simulink model "open_model"  (R2021b)
settings: Solver=ode45  StartTime=0.0  StopTime=3600*60*24  RelTol=1e-6
values from neighbouring files (symbols this model uses):
  alpha = 3.7541    [Parameters.m]
  beta = beta/(24*60*60)    (= 1.57476851852e-05)    [Parameters.m]
  dI = dI/(24*60*60)    (= 1.15740740741e-06)    [Parameters.m]
  dV = dV/(24*60*60)    (= 2.13148148148e-05)    [Parameters.m]
  I0 = 0    [Parameters.m]
  L = 936.4293    [Parameters.m]
  r = r/(24*60*60)    (= 6.97916666667e-07)    [Parameters.m]
  S0 = 128.1481    [Parameters.m]
  V0 = 0    [Parameters.m]
undefined symbols (not defined in the file or in its folder): sigbuilder_block
settings Model: Creator=zceexc1  LastModifiedBy=chenx
settings DebuggingCC: UnconnectedInputMsg=none  UnconnectedOutputMsg=none  UnconnectedLineMsg=none
settings RTWCC: DLArmComputeVersion=20.02.1

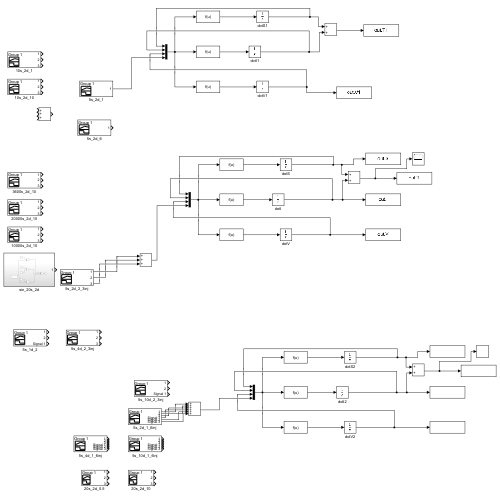
[thumbnail: Simulink's stored preview of the top-level diagram]
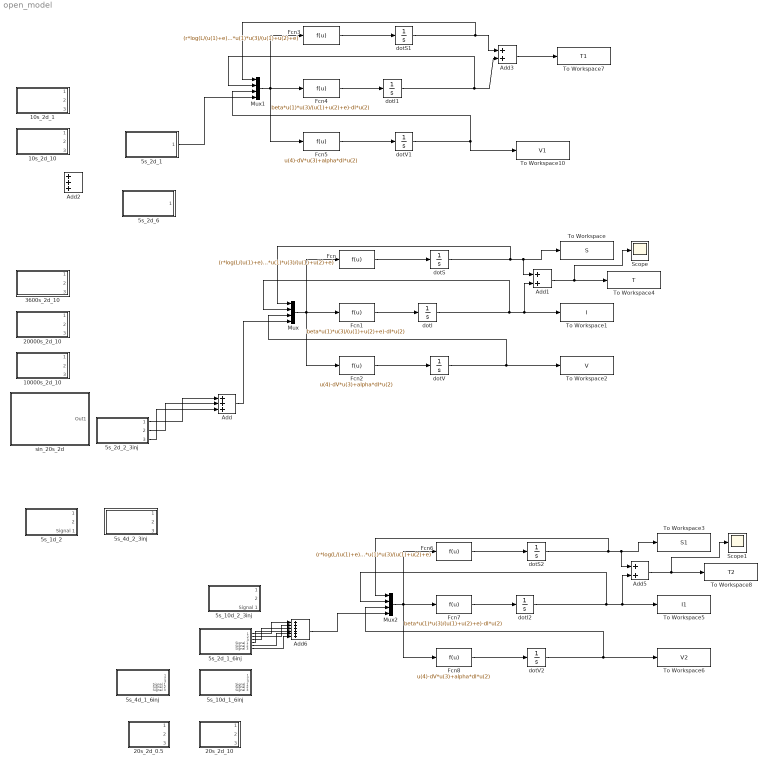
== system open_model ==
  10000s_2d_10 : Subsystem  Tag=STV Subsys  LoadFcn=sigbuilder_block('load');  StartFcn=sigbuilder_block('start');  StopFcn=sigbuilder_block('stop');  ClipboardFcn=sigbuilder_block('clipboard');  mask(Sigbuilder block){tuvar=[0:10]}
      mask help: Simulink:masks:SigbuilderBlock_MD
      mask init:
      | if ~strcmp(get_param(bdroot(gcbh),'SimulationStatus'),'stopped') tuvar = sigbuilder_block('maskInit'); end
      settings: CopyFcn=sigbuilder_block('copy');  DeleteFcn=sigbuilder_block('delete');  ModelCloseFcn=sigbuilder_block('modelClose');  PreSaveFcn=sigbuilder_block('preSave');  PauseFcn=sigbuilder_block('pause');  ContinueFcn=sigbuilder_block('continue');  NameChangeFcn=sigbuilder_block('namechange');  OpenFcn=sigbuilder_block('open',[190.5 88.5 550.5 362.5 ]);  CloseFcn=sigbuilder_block('close');
      mask Display: plot(0, 0, 100, 100,[2, 2, 32, 32, 2], [68, 8, 8, 68, 68],[32, 2], [38, 38], [32, 19, 2],[53, 60, 44], [32, 17, 17, 2],[16, 16, 31, 31]);txt = getActiveGroup(gcbh);text(2, 100, txt,'verticalAlignment', 'top');
  10s_2d_1 : Subsystem  Tag=STV Subsys  LoadFcn=sigbuilder_block('load');  StartFcn=sigbuilder_block('start');  StopFcn=sigbuilder_block('stop');  ClipboardFcn=sigbuilder_block('clipboard');  mask(Sigbuilder block){tuvar=[0:10]}
      mask help: Simulink:masks:SigbuilderBlock_MD
      mask init:
      | if ~strcmp(get_param(bdroot(gcbh),'SimulationStatus'),'stopped') tuvar = sigbuilder_block('maskInit'); end
      settings: CopyFcn=sigbuilder_block('copy');  DeleteFcn=sigbuilder_block('delete');  ModelCloseFcn=sigbuilder_block('modelClose');  PreSaveFcn=sigbuilder_block('preSave');  PauseFcn=sigbuilder_block('pause');  ContinueFcn=sigbuilder_block('continue');  NameChangeFcn=sigbuilder_block('namechange');  OpenFcn=sigbuilder_block('open',[190.5 88.5 550.5 362.5 ]);  CloseFcn=sigbuilder_block('close');
      mask Display: plot(0, 0, 100, 100,[2, 2, 32, 32, 2], [68, 8, 8, 68, 68],[32, 2], [38, 38], [32, 19, 2],[53, 60, 44], [32, 17, 17, 2],[16, 16, 31, 31]);txt = getActiveGroup(gcbh);text(2, 100, txt,'verticalAlignment', 'top');
  10s_2d_10 : Subsystem  Tag=STV Subsys  LoadFcn=sigbuilder_block('load');  StartFcn=sigbuilder_block('start');  StopFcn=sigbuilder_block('stop');  ClipboardFcn=sigbuilder_block('clipboard');  mask(Sigbuilder block){tuvar=[0:10]}
      mask help: Simulink:masks:SigbuilderBlock_MD
      mask init:
      | if ~strcmp(get_param(bdroot(gcbh),'SimulationStatus'),'stopped') tuvar = sigbuilder_block('maskInit'); end
      settings: CopyFcn=sigbuilder_block('copy');  DeleteFcn=sigbuilder_block('delete');  ModelCloseFcn=sigbuilder_block('modelClose');  PreSaveFcn=sigbuilder_block('preSave');  PauseFcn=sigbuilder_block('pause');  ContinueFcn=sigbuilder_block('continue');  NameChangeFcn=sigbuilder_block('namechange');  OpenFcn=sigbuilder_block('open',[190.5 88.5 550.5 362.5 ]);  CloseFcn=sigbuilder_block('close');
      mask Display: plot(0, 0, 100, 100,[2, 2, 32, 32, 2], [68, 8, 8, 68, 68],[32, 2], [38, 38], [32, 19, 2],[53, 60, 44], [32, 17, 17, 2],[16, 16, 31, 31]);txt = getActiveGroup(gcbh);text(2, 100, txt,'verticalAlignment', 'top');
  20000s_2d_10 : Subsystem  Tag=STV Subsys  LoadFcn=sigbuilder_block('load');  StartFcn=sigbuilder_block('start');  StopFcn=sigbuilder_block('stop');  ClipboardFcn=sigbuilder_block('clipboard');  mask(Sigbuilder block){tuvar=[0:10]}
      mask help: Simulink:masks:SigbuilderBlock_MD
      mask init:
      | if ~strcmp(get_param(bdroot(gcbh),'SimulationStatus'),'stopped') tuvar = sigbuilder_block('maskInit'); end
      settings: CopyFcn=sigbuilder_block('copy');  DeleteFcn=sigbuilder_block('delete');  ModelCloseFcn=sigbuilder_block('modelClose');  PreSaveFcn=sigbuilder_block('preSave');  PauseFcn=sigbuilder_block('pause');  ContinueFcn=sigbuilder_block('continue');  NameChangeFcn=sigbuilder_block('namechange');  OpenFcn=sigbuilder_block('open',[190.5 88.5 550.5 362.5 ]);  CloseFcn=sigbuilder_block('close');
      mask Display: plot(0, 0, 100, 100,[2, 2, 32, 32, 2], [68, 8, 8, 68, 68],[32, 2], [38, 38], [32, 19, 2],[53, 60, 44], [32, 17, 17, 2],[16, 16, 31, 31]);txt = getActiveGroup(gcbh);text(2, 100, txt,'verticalAlignment', 'top');
  20s_2d_0.5 : Subsystem  Tag=STV Subsys  LoadFcn=sigbuilder_block('load');  StartFcn=sigbuilder_block('start');  StopFcn=sigbuilder_block('stop');  ClipboardFcn=sigbuilder_block('clipboard');  mask(Sigbuilder block){tuvar=[0:10]}
      mask help: Simulink:masks:SigbuilderBlock_MD
      mask init:
      | if ~strcmp(get_param(bdroot(gcbh),'SimulationStatus'),'stopped') tuvar = sigbuilder_block('maskInit'); end
      settings: CopyFcn=sigbuilder_block('copy');  DeleteFcn=sigbuilder_block('delete');  ModelCloseFcn=sigbuilder_block('modelClose');  PreSaveFcn=sigbuilder_block('preSave');  PauseFcn=sigbuilder_block('pause');  ContinueFcn=sigbuilder_block('continue');  NameChangeFcn=sigbuilder_block('namechange');  OpenFcn=sigbuilder_block('open',[190.5 88.5 550.5 362.5 ]);  CloseFcn=sigbuilder_block('close');
      mask Display: plot(0, 0, 100, 100,[2, 2, 32, 32, 2], [68, 8, 8, 68, 68],[32, 2], [38, 38], [32, 19, 2],[53, 60, 44], [32, 17, 17, 2],[16, 16, 31, 31]);txt = getActiveGroup(gcbh);text(2, 100, txt,'verticalAlignment', 'top');
  20s_2d_10 : Subsystem  Tag=STV Subsys  LoadFcn=sigbuilder_block('load');  StartFcn=sigbuilder_block('start');  StopFcn=sigbuilder_block('stop');  ClipboardFcn=sigbuilder_block('clipboard');  mask(Sigbuilder block){tuvar=[0:10]}
      mask help: Simulink:masks:SigbuilderBlock_MD
      mask init:
      | if ~strcmp(get_param(bdroot(gcbh),'SimulationStatus'),'stopped') tuvar = sigbuilder_block('maskInit'); end
      settings: CopyFcn=sigbuilder_block('copy');  DeleteFcn=sigbuilder_block('delete');  ModelCloseFcn=sigbuilder_block('modelClose');  PreSaveFcn=sigbuilder_block('preSave');  PauseFcn=sigbuilder_block('pause');  ContinueFcn=sigbuilder_block('continue');  NameChangeFcn=sigbuilder_block('namechange');  OpenFcn=sigbuilder_block('open',[190.5 88.5 550.5 362.5 ]);  CloseFcn=sigbuilder_block('close');
      mask Display: plot(0, 0, 100, 100,[2, 2, 32, 32, 2], [68, 8, 8, 68, 68],[32, 2], [38, 38], [32, 19, 2],[53, 60, 44], [32, 17, 17, 2],[16, 16, 31, 31]);txt = getActiveGroup(gcbh);text(2, 100, txt,'verticalAlignment', 'top');
  3600s_2d_10 : Subsystem  Tag=STV Subsys  LoadFcn=sigbuilder_block('load');  StartFcn=sigbuilder_block('start');  StopFcn=sigbuilder_block('stop');  ClipboardFcn=sigbuilder_block('clipboard');  mask(Sigbuilder block){tuvar=[0:10]}
      mask help: Simulink:masks:SigbuilderBlock_MD
      mask init:
      | if ~strcmp(get_param(bdroot(gcbh),'SimulationStatus'),'stopped') tuvar = sigbuilder_block('maskInit'); end
      settings: CopyFcn=sigbuilder_block('copy');  DeleteFcn=sigbuilder_block('delete');  ModelCloseFcn=sigbuilder_block('modelClose');  PreSaveFcn=sigbuilder_block('preSave');  PauseFcn=sigbuilder_block('pause');  ContinueFcn=sigbuilder_block('continue');  NameChangeFcn=sigbuilder_block('namechange');  OpenFcn=sigbuilder_block('open',[190.5 88.5 550.5 362.5 ]);  CloseFcn=sigbuilder_block('close');
      mask Display: plot(0, 0, 100, 100,[2, 2, 32, 32, 2], [68, 8, 8, 68, 68],[32, 2], [38, 38], [32, 19, 2],[53, 60, 44], [32, 17, 17, 2],[16, 16, 31, 31]);txt = getActiveGroup(gcbh);text(2, 100, txt,'verticalAlignment', 'top');
  5s_10d_1_6inj : Subsystem  Tag=STV Subsys  LoadFcn=sigbuilder_block('load');  StartFcn=sigbuilder_block('start');  StopFcn=sigbuilder_block('stop');  ClipboardFcn=sigbuilder_block('clipboard');  mask(Sigbuilder block){tuvar=[0:10]}
      mask help: Simulink:masks:SigbuilderBlock_MD
      mask init:
      | if ~strcmp(get_param(bdroot(gcbh),'SimulationStatus'),'stopped') tuvar = sigbuilder_block('maskInit'); end
      settings: CopyFcn=sigbuilder_block('copy');  DeleteFcn=sigbuilder_block('delete');  ModelCloseFcn=sigbuilder_block('modelClose');  PreSaveFcn=sigbuilder_block('preSave');  PauseFcn=sigbuilder_block('pause');  ContinueFcn=sigbuilder_block('continue');  NameChangeFcn=sigbuilder_block('namechange');  OpenFcn=sigbuilder_block('open',[190.5 88.5 550.5 362.5 ]);  CloseFcn=sigbuilder_block('close');
      mask Display: plot(0, 0, 100, 100,[2, 2, 32, 32, 2], [68, 8, 8, 68, 68],[32, 2], [38, 38], [32, 19, 2],[53, 60, 44], [32, 17, 17, 2],[16, 16, 31, 31]);txt = getActiveGroup(gcbh);text(2, 100, txt,'verticalAlignment', 'top');
  5s_10d_2_3inj : Subsystem  Tag=STV Subsys  LoadFcn=sigbuilder_block('load');  StartFcn=sigbuilder_block('start');  StopFcn=sigbuilder_block('stop');  ClipboardFcn=sigbuilder_block('clipboard');  mask(Sigbuilder block){tuvar=[0:10]}
      mask help: Simulink:masks:SigbuilderBlock_MD
      mask init:
      | if ~strcmp(get_param(bdroot(gcbh),'SimulationStatus'),'stopped') tuvar = sigbuilder_block('maskInit'); end
      settings: CopyFcn=sigbuilder_block('copy');  DeleteFcn=sigbuilder_block('delete');  ModelCloseFcn=sigbuilder_block('modelClose');  PreSaveFcn=sigbuilder_block('preSave');  PauseFcn=sigbuilder_block('pause');  ContinueFcn=sigbuilder_block('continue');  NameChangeFcn=sigbuilder_block('namechange');  OpenFcn=sigbuilder_block('open',[190.5 88.5 550.5 362.5 ]);  CloseFcn=sigbuilder_block('close');
      mask Display: plot(0, 0, 100, 100,[2, 2, 32, 32, 2], [68, 8, 8, 68, 68],[32, 2], [38, 38], [32, 19, 2],[53, 60, 44], [32, 17, 17, 2],[16, 16, 31, 31]);txt = getActiveGroup(gcbh);text(2, 100, txt,'verticalAlignment', 'top');
  5s_1d_2 : Subsystem  Tag=STV Subsys  LoadFcn=sigbuilder_block('load');  StartFcn=sigbuilder_block('start');  StopFcn=sigbuilder_block('stop');  ClipboardFcn=sigbuilder_block('clipboard');  mask(Sigbuilder block){tuvar=[0:10]}
      mask help: Simulink:masks:SigbuilderBlock_MD
      mask init:
      | if ~strcmp(get_param(bdroot(gcbh),'SimulationStatus'),'stopped') tuvar = sigbuilder_block('maskInit'); end
      settings: CopyFcn=sigbuilder_block('copy');  DeleteFcn=sigbuilder_block('delete');  ModelCloseFcn=sigbuilder_block('modelClose');  PreSaveFcn=sigbuilder_block('preSave');  PauseFcn=sigbuilder_block('pause');  ContinueFcn=sigbuilder_block('continue');  NameChangeFcn=sigbuilder_block('namechange');  OpenFcn=sigbuilder_block('open',[190.5 88.5 550.5 362.5 ]);  CloseFcn=sigbuilder_block('close');
      mask Display: plot(0, 0, 100, 100,[2, 2, 32, 32, 2], [68, 8, 8, 68, 68],[32, 2], [38, 38], [32, 19, 2],[53, 60, 44], [32, 17, 17, 2],[16, 16, 31, 31]);txt = getActiveGroup(gcbh);text(2, 100, txt,'verticalAlignment', 'top');
  5s_2d_1 : Subsystem  Tag=STV Subsys  LoadFcn=sigbuilder_block('load');  StartFcn=sigbuilder_block('start');  StopFcn=sigbuilder_block('stop');  ClipboardFcn=sigbuilder_block('clipboard');  mask(Sigbuilder block){tuvar=[0:10]}
      mask help: Simulink:masks:SigbuilderBlock_MD
      mask init:
      | if ~strcmp(get_param(bdroot(gcbh),'SimulationStatus'),'stopped') tuvar = sigbuilder_block('maskInit'); end
      settings: CopyFcn=sigbuilder_block('copy');  DeleteFcn=sigbuilder_block('delete');  ModelCloseFcn=sigbuilder_block('modelClose');  PreSaveFcn=sigbuilder_block('preSave');  PauseFcn=sigbuilder_block('pause');  ContinueFcn=sigbuilder_block('continue');  NameChangeFcn=sigbuilder_block('namechange');  OpenFcn=sigbuilder_block('open',[190.5 88.5 550.5 362.5 ]);  CloseFcn=sigbuilder_block('close');
      mask Display: plot(0, 0, 100, 100,[2, 2, 32, 32, 2], [68, 8, 8, 68, 68],[32, 2], [38, 38], [32, 19, 2],[53, 60, 44], [32, 17, 17, 2],[16, 16, 31, 31]);txt = getActiveGroup(gcbh);text(2, 100, txt,'verticalAlignment', 'top');
  5s_2d_1_6inj : Subsystem  Tag=STV Subsys  LoadFcn=sigbuilder_block('load');  StartFcn=sigbuilder_block('start');  StopFcn=sigbuilder_block('stop');  ClipboardFcn=sigbuilder_block('clipboard');  mask(Sigbuilder block){tuvar=[0:10]}
      mask help: Simulink:masks:SigbuilderBlock_MD
      mask init:
      | if ~strcmp(get_param(bdroot(gcbh),'SimulationStatus'),'stopped') tuvar = sigbuilder_block('maskInit'); end
      settings: CopyFcn=sigbuilder_block('copy');  DeleteFcn=sigbuilder_block('delete');  ModelCloseFcn=sigbuilder_block('modelClose');  PreSaveFcn=sigbuilder_block('preSave');  PauseFcn=sigbuilder_block('pause');  ContinueFcn=sigbuilder_block('continue');  NameChangeFcn=sigbuilder_block('namechange');  OpenFcn=sigbuilder_block('open',[190.5 88.5 550.5 362.5 ]);  CloseFcn=sigbuilder_block('close');
      mask Display: plot(0, 0, 100, 100,[2, 2, 32, 32, 2], [68, 8, 8, 68, 68],[32, 2], [38, 38], [32, 19, 2],[53, 60, 44], [32, 17, 17, 2],[16, 16, 31, 31]);txt = getActiveGroup(gcbh);text(2, 100, txt,'verticalAlignment', 'top');
  5s_2d_2_3inj : Subsystem  Tag=STV Subsys  LoadFcn=sigbuilder_block('load');  StartFcn=sigbuilder_block('start');  StopFcn=sigbuilder_block('stop');  ClipboardFcn=sigbuilder_block('clipboard');  mask(Sigbuilder block){tuvar=[0:10]}
      mask help: Simulink:masks:SigbuilderBlock_MD
      mask init:
      | if ~strcmp(get_param(bdroot(gcbh),'SimulationStatus'),'stopped') tuvar = sigbuilder_block('maskInit'); end
      settings: CopyFcn=sigbuilder_block('copy');  DeleteFcn=sigbuilder_block('delete');  ModelCloseFcn=sigbuilder_block('modelClose');  PreSaveFcn=sigbuilder_block('preSave');  PauseFcn=sigbuilder_block('pause');  ContinueFcn=sigbuilder_block('continue');  NameChangeFcn=sigbuilder_block('namechange');  OpenFcn=sigbuilder_block('open',[190.5 88.5 550.5 362.5 ]);  CloseFcn=sigbuilder_block('close');
      mask Display: plot(0, 0, 100, 100,[2, 2, 32, 32, 2], [68, 8, 8, 68, 68],[32, 2], [38, 38], [32, 19, 2],[53, 60, 44], [32, 17, 17, 2],[16, 16, 31, 31]);txt = getActiveGroup(gcbh);text(2, 100, txt,'verticalAlignment', 'top');
  5s_2d_6 : Subsystem  Tag=STV Subsys  LoadFcn=sigbuilder_block('load');  StartFcn=sigbuilder_block('start');  StopFcn=sigbuilder_block('stop');  ClipboardFcn=sigbuilder_block('clipboard');  mask(Sigbuilder block){tuvar=[0:10]}
      mask help: Simulink:masks:SigbuilderBlock_MD
      mask init:
      | if ~strcmp(get_param(bdroot(gcbh),'SimulationStatus'),'stopped') tuvar = sigbuilder_block('maskInit'); end
      settings: CopyFcn=sigbuilder_block('copy');  DeleteFcn=sigbuilder_block('delete');  ModelCloseFcn=sigbuilder_block('modelClose');  PreSaveFcn=sigbuilder_block('preSave');  PauseFcn=sigbuilder_block('pause');  ContinueFcn=sigbuilder_block('continue');  NameChangeFcn=sigbuilder_block('namechange');  OpenFcn=sigbuilder_block('open',[190.5 88.5 550.5 362.5 ]);  CloseFcn=sigbuilder_block('close');
      mask Display: plot(0, 0, 100, 100,[2, 2, 32, 32, 2], [68, 8, 8, 68, 68],[32, 2], [38, 38], [32, 19, 2],[53, 60, 44], [32, 17, 17, 2],[16, 16, 31, 31]);txt = getActiveGroup(gcbh);text(2, 100, txt,'verticalAlignment', 'top');
  5s_4d_1_6inj : Subsystem  Tag=STV Subsys  LoadFcn=sigbuilder_block('load');  StartFcn=sigbuilder_block('start');  StopFcn=sigbuilder_block('stop');  ClipboardFcn=sigbuilder_block('clipboard');  mask(Sigbuilder block){tuvar=[0:10]}
      mask help: Simulink:masks:SigbuilderBlock_MD
      mask init:
      | if ~strcmp(get_param(bdroot(gcbh),'SimulationStatus'),'stopped') tuvar = sigbuilder_block('maskInit'); end
      settings: CopyFcn=sigbuilder_block('copy');  DeleteFcn=sigbuilder_block('delete');  ModelCloseFcn=sigbuilder_block('modelClose');  PreSaveFcn=sigbuilder_block('preSave');  PauseFcn=sigbuilder_block('pause');  ContinueFcn=sigbuilder_block('continue');  NameChangeFcn=sigbuilder_block('namechange');  OpenFcn=sigbuilder_block('open',[190.5 88.5 550.5 362.5 ]);  CloseFcn=sigbuilder_block('close');
      mask Display: plot(0, 0, 100, 100,[2, 2, 32, 32, 2], [68, 8, 8, 68, 68],[32, 2], [38, 38], [32, 19, 2],[53, 60, 44], [32, 17, 17, 2],[16, 16, 31, 31]);txt = getActiveGroup(gcbh);text(2, 100, txt,'verticalAlignment', 'top');
  5s_4d_2_3inj : Subsystem  Tag=STV Subsys  LoadFcn=sigbuilder_block('load');  StartFcn=sigbuilder_block('start');  StopFcn=sigbuilder_block('stop');  ClipboardFcn=sigbuilder_block('clipboard');  mask(Sigbuilder block){tuvar=[0:10]}
      mask help: Simulink:masks:SigbuilderBlock_MD
      mask init:
      | if ~strcmp(get_param(bdroot(gcbh),'SimulationStatus'),'stopped') tuvar = sigbuilder_block('maskInit'); end
      settings: CopyFcn=sigbuilder_block('copy');  DeleteFcn=sigbuilder_block('delete');  ModelCloseFcn=sigbuilder_block('modelClose');  PreSaveFcn=sigbuilder_block('preSave');  PauseFcn=sigbuilder_block('pause');  ContinueFcn=sigbuilder_block('continue');  NameChangeFcn=sigbuilder_block('namechange');  OpenFcn=sigbuilder_block('open',[190.5 88.5 550.5 362.5 ]);  CloseFcn=sigbuilder_block('close');
      mask Display: plot(0, 0, 100, 100,[2, 2, 32, 32, 2], [68, 8, 8, 68, 68],[32, 2], [38, 38], [32, 19, 2],[53, 60, 44], [32, 17, 17, 2],[16, 16, 31, 31]);txt = getActiveGroup(gcbh);text(2, 100, txt,'verticalAlignment', 'top');
  Add : Sum  Inputs=+++
  Add1 : Sum
  Add2 : Sum  Inputs=+++
  Add3 : Sum
  Add5 : Sum
  Add6 : Sum  Inputs=++++++
  Fcn : Fcn  Expr=(r*log(L/(u(1)+e)))*u(1)-beta*u(1)*u(3)/(u(1)+u(2)+e)
  Fcn1 : Fcn  Expr=beta*u(1)*u(3)/(u(1)+u(2)+e)-dI*u(2)
  Fcn2 : Fcn  Expr=u(4)-dV*u(3)+alpha*dI*u(2)
  Fcn3 : Fcn  Expr=(r*log(L/(u(1)+e)))*u(1)-beta*u(1)*u(3)/(u(1)+u(2)+e)
  Fcn4 : Fcn  Expr=beta*u(1)*u(3)/(u(1)+u(2)+e)-dI*u(2)
  Fcn5 : Fcn  Expr=u(4)-dV*u(3)+alpha*dI*u(2)
  Fcn6 : Fcn  Expr=(r*log(L/(u(1)+e)))*u(1)-beta*u(1)*u(3)/(u(1)+u(2)+e)
  Fcn7 : Fcn  Expr=beta*u(1)*u(3)/(u(1)+u(2)+e)-dI*u(2)
  Fcn8 : Fcn  Expr=u(4)-dV*u(3)+alpha*dI*u(2)
  Mux : Mux
  Mux1 : Mux
  Mux2 : Mux
  Scope : Scope
  Scope1 : Scope
  To Workspace : ToWorkspace  VariableName=S  SampleTime=-1
  To Workspace1 : ToWorkspace  VariableName=I  SampleTime=-1
  To Workspace10 : ToWorkspace  VariableName=V1  SampleTime=-1
  To Workspace2 : ToWorkspace  VariableName=V  SampleTime=-1
  To Workspace3 : ToWorkspace  VariableName=S1  SampleTime=-1
  To Workspace4 : ToWorkspace  VariableName=T  SampleTime=-1
  To Workspace5 : ToWorkspace  VariableName=I1  SampleTime=-1
  To Workspace6 : ToWorkspace  VariableName=V2  SampleTime=-1
  To Workspace7 : ToWorkspace  VariableName=T1  SampleTime=-1
  To Workspace8 : ToWorkspace  VariableName=T2  SampleTime=-1
  dotI : Integrator  InitialCondition=I0
  dotI1 : Integrator  InitialCondition=I0
  dotI2 : Integrator  InitialCondition=I0
  dotS : Integrator  InitialCondition=S0
  dotS1 : Integrator  InitialCondition=S0
  dotS2 : Integrator  InitialCondition=S0
  dotV : Integrator  InitialCondition=V0
  dotV1 : Integrator  InitialCondition=V0
  dotV2 : Integrator  InitialCondition=V0
  sin_20s_2d : Subsystem
  wires:
  Fcn/1 -> dotS/1
  Fcn1/1 -> dotI/1
  Fcn2/1 -> dotV/1
  dotV/1 -> Mux/3, To Workspace2/1
  dotS/1 -> Add1/1, To Workspace/1, Mux/1
  dotI/1 -> Add1/2, To Workspace1/1, Mux/2
  Mux/1 -> Fcn1/1, Fcn/1, Fcn2/1
  Add/1 -> Mux/4
  Add1/1 -> Scope/1, To Workspace4/1
  Mux1/1 -> Fcn4/1, Fcn3/1, Fcn5/1
  dotV1/1 -> Mux1/3, To Workspace10/1
  Fcn5/1 -> dotV1/1
  Fcn4/1 -> dotI1/1
  Add3/1 -> To Workspace7/1
  dotS1/1 -> Add3/1, Mux1/1
  Fcn3/1 -> dotS1/1
  dotI1/1 -> Add3/2, Mux1/2
  Mux2/1 -> Fcn7/1, Fcn6/1, Fcn8/1
  dotV2/1 -> Mux2/3, To Workspace6/1
  Fcn8/1 -> dotV2/1
  Fcn7/1 -> dotI2/1
  Add5/1 -> Scope1/1, To Workspace8/1
  dotS2/1 -> Add5/1, To Workspace3/1, Mux2/1
  Fcn6/1 -> dotS2/1
  dotI2/1 -> Add5/2, To Workspace5/1, Mux2/2
  Add6/1 -> Mux2/4
  5s_2d_1_6inj/1(1) -> Add6/1
  5s_2d_1_6inj/2(2) -> Add6/2
  5s_2d_1_6inj/3(3) -> Add6/3
  5s_2d_1_6inj/4(Signal 1) -> Add6/4
  5s_2d_1_6inj/5(Signal 2) -> Add6/5
  5s_2d_1_6inj/6(Signal 3) -> Add6/6
  5s_2d_2_3inj/1(1) -> Add/1
  5s_2d_2_3inj/2(2) -> Add/2
  5s_2d_2_3inj/3(3) -> Add/3
  5s_2d_1/1(1) -> Mux1/4

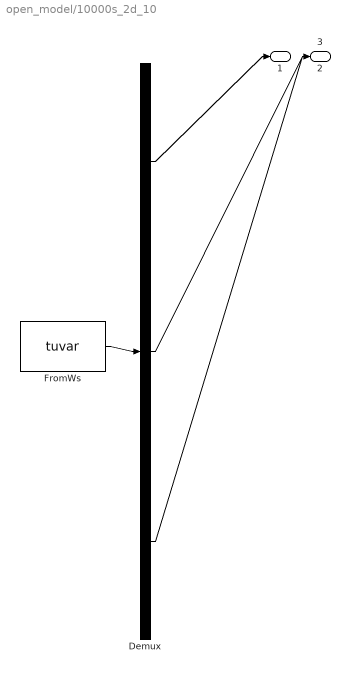
== system open_model/10000s_2d_10 ==
  Demux : Demux  Tag=STV Demux  Outputs=3
      settings: DisplayOption=none
  FromWs : FromWorkspace  Tag=STV FromWs  VariableName=tuvar
      SigBuilderData=|
      | common.afterFinalStr = 'Extrapolate'
      | common.sampleTime = 0
      | dataSet.timeRange = [0 864000]
      | dataSet.name = 'Group 1'
      | sbobj.Groups.Name = 'Group 1'
      | sbobj.Groups.Signals(1).Name = '1'
      | sbobj.Groups.Signals(1).XData = [0 10000 10000 864000]
      | sbobj.Groups.Signals(1).YData = [10 10 0 0]
      | sbobj.Groups.Signals(2).Name = '2'
      | sbobj.Groups.Signals(2).XData = [0 172800 172800 182800 182800 864000]
      | sbobj.Groups.Signals(2).YData = [0 0 10 10 0 0]
      | sbobj.Groups.Signals(3).Name = '3'
      | sbobj.Groups.Signals(3).XData = [0 345600 345600 355600 355600 864000]
      | sbobj.Groups.Signals(3).YData = [0 0 10 10 0 0]
      | sbobj.Groups.TimeRange = [0 864000]
  1 : Outport  Tag=STV Outport
  2 : Outport  Tag=STV Outport  Port=2
  3 : Outport  Tag=STV Outport  Port=3
  wires:
  Demux/1 -> 1/1
  Demux/2 -> 2/1
  Demux/3 -> 3/1
  FromWs/1 -> Demux/1

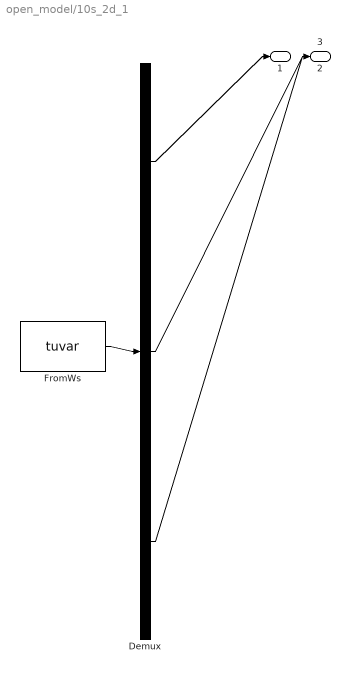
== system open_model/10s_2d_1 ==
  Demux : Demux  Tag=STV Demux  Outputs=3
      settings: DisplayOption=none
  FromWs : FromWorkspace  Tag=STV FromWs  VariableName=tuvar
      SigBuilderData=|
      | common.afterFinalStr = 'Extrapolate'
      | common.sampleTime = 0
      | dataSet.timeRange = [0 864000]
      | dataSet.name = 'Group 1'
      | sbobj.Groups.Name = 'Group 1'
      | sbobj.Groups.Signals(1).Name = '1'
      | sbobj.Groups.Signals(1).XData = [0 10 10 864000]
      | sbobj.Groups.Signals(1).YData = [1 1 0 0]
      | sbobj.Groups.Signals(2).Name = '2'
      | sbobj.Groups.Signals(2).XData = [0 172800 172800 172810 172810 864000]
      | sbobj.Groups.Signals(2).YData = [0 0 1 1 0 0]
      | sbobj.Groups.Signals(3).Name = '3'
      | sbobj.Groups.Signals(3).XData = [0 345600 345600 345610 345610 864000]
      | sbobj.Groups.Signals(3).YData = [0 0 1 1 0 0]
      | sbobj.Groups.TimeRange = [0 864000]
  1 : Outport  Tag=STV Outport
  2 : Outport  Tag=STV Outport  Port=2
  3 : Outport  Tag=STV Outport  Port=3
  wires:
  FromWs/1 -> Demux/1
  Demux/3 -> 3/1
  Demux/2 -> 2/1
  Demux/1 -> 1/1

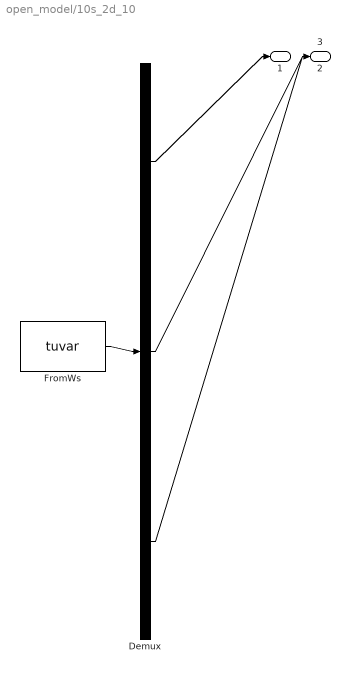
== system open_model/10s_2d_10 ==
  Demux : Demux  Tag=STV Demux  Outputs=3
      settings: DisplayOption=none
  FromWs : FromWorkspace  Tag=STV FromWs  VariableName=tuvar
      SigBuilderData=|
      | common.afterFinalStr = 'Extrapolate'
      | common.sampleTime = 0
      | dataSet.timeRange = [0 864000]
      | dataSet.name = 'Group 1'
      | sbobj.Groups.Name = 'Group 1'
      | sbobj.Groups.Signals(1).Name = '1'
      | sbobj.Groups.Signals(1).XData = [0 10 10 864000]
      | sbobj.Groups.Signals(1).YData = [10 10 0 0]
      | sbobj.Groups.Signals(2).Name = '2'
      | sbobj.Groups.Signals(2).XData = [0 172800 172800 172810 172810 864000]
      | sbobj.Groups.Signals(2).YData = [0 0 10 10 0 0]
      | sbobj.Groups.Signals(3).Name = '3'
      | sbobj.Groups.Signals(3).XData = [0 345600 345600 345610 345610 864000]
      | sbobj.Groups.Signals(3).YData = [0 0 10 10 0 0]
      | sbobj.Groups.TimeRange = [0 864000]
  1 : Outport  Tag=STV Outport
  2 : Outport  Tag=STV Outport  Port=2
  3 : Outport  Tag=STV Outport  Port=3
  wires:
  Demux/1 -> 1/1
  Demux/2 -> 2/1
  Demux/3 -> 3/1
  FromWs/1 -> Demux/1

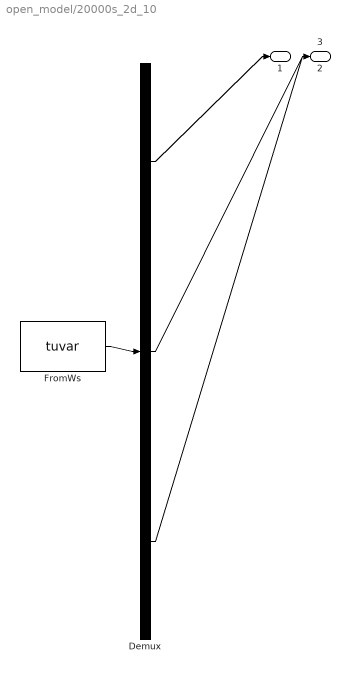
== system open_model/20000s_2d_10 ==
  Demux : Demux  Tag=STV Demux  Outputs=3
      settings: DisplayOption=none
  FromWs : FromWorkspace  Tag=STV FromWs  VariableName=tuvar
      SigBuilderData=|
      | common.afterFinalStr = 'Extrapolate'
      | common.sampleTime = 0
      | dataSet.timeRange = [0 864000]
      | dataSet.name = 'Group 1'
      | sbobj.Groups.Name = 'Group 1'
      | sbobj.Groups.Signals(1).Name = '1'
      | sbobj.Groups.Signals(1).XData = [0 20000 20000 864000]
      | sbobj.Groups.Signals(1).YData = [10 10 0 0]
      | sbobj.Groups.Signals(2).Name = '2'
      | sbobj.Groups.Signals(2).XData = [0 172800 172800 192800 192800 864000]
      | sbobj.Groups.Signals(2).YData = [0 0 10 10 0 0]
      | sbobj.Groups.Signals(3).Name = '3'
      | sbobj.Groups.Signals(3).XData = [0 345600 345600 365600 365600 864000]
      | sbobj.Groups.Signals(3).YData = [0 0 10 10 0 0]
      | sbobj.Groups.TimeRange = [0 864000]
  1 : Outport  Tag=STV Outport
  2 : Outport  Tag=STV Outport  Port=2
  3 : Outport  Tag=STV Outport  Port=3
  wires:
  Demux/1 -> 1/1
  Demux/2 -> 2/1
  Demux/3 -> 3/1
  FromWs/1 -> Demux/1

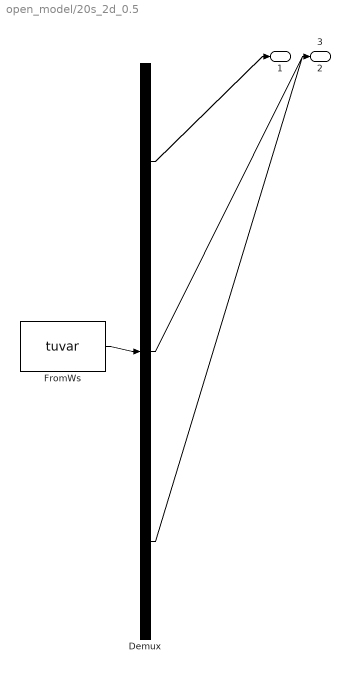
== system open_model/20s_2d_0.5 ==
  Demux : Demux  Tag=STV Demux  Outputs=3
      settings: DisplayOption=none
  FromWs : FromWorkspace  Tag=STV FromWs  VariableName=tuvar
      SigBuilderData=|
      | common.afterFinalStr = 'Extrapolate'
      | common.sampleTime = 0
      | dataSet.timeRange = [0 5184000]
      | dataSet.name = 'Group 1'
      | sbobj.Groups.Name = 'Group 1'
      | sbobj.Groups.Signals(1).Name = '1'
      | sbobj.Groups.Signals(1).XData = [0 20 20 5184000]
      | sbobj.Groups.Signals(1).YData = [0.49 0.5 0 0]
      | sbobj.Groups.Signals(2).Name = '2'
      | sbobj.Groups.Signals(2).XData = [0 172800 172800 172820 172820 5184000]
      | sbobj.Groups.Signals(2).YData = [0 0 0.5 0.5 0 0]
      | sbobj.Groups.Signals(3).Name = '3'
      | sbobj.Groups.Signals(3).XData = [0 345600 345600 345620 345620 5184000]
      | sbobj.Groups.Signals(3).YData = [0 0 0.5 0.5 0 0]
      | sbobj.Groups.TimeRange = [0 5184000]
  1 : Outport  Tag=STV Outport
  2 : Outport  Tag=STV Outport  Port=2
  3 : Outport  Tag=STV Outport  Port=3
  wires:
  Demux/1 -> 1/1
  Demux/2 -> 2/1
  Demux/3 -> 3/1
  FromWs/1 -> Demux/1

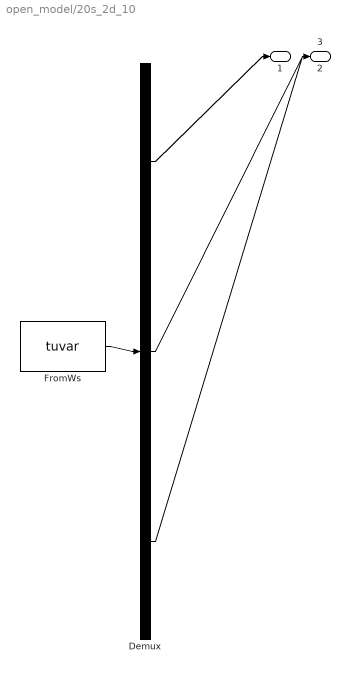
== system open_model/20s_2d_10 ==
  Demux : Demux  Tag=STV Demux  Outputs=3
      settings: DisplayOption=none
  FromWs : FromWorkspace  Tag=STV FromWs  VariableName=tuvar
      SigBuilderData=|
      | common.afterFinalStr = 'Extrapolate'
      | common.sampleTime = 0
      | dataSet.timeRange = [0 5184000]
      | dataSet.name = 'Group 1'
      | sbobj.Groups.Name = 'Group 1'
      | sbobj.Groups.Signals(1).Name = '1'
      | sbobj.Groups.Signals(1).XData = [0 20 20 5184000]
      | sbobj.Groups.Signals(1).YData = [10 10 0 0]
      | sbobj.Groups.Signals(2).Name = '2'
      | sbobj.Groups.Signals(2).XData = [0 172800 172800 172820 172820 5184000]
      | sbobj.Groups.Signals(2).YData = [0 0 10 10 0 0]
      | sbobj.Groups.Signals(3).Name = '3'
      | sbobj.Groups.Signals(3).XData = [0 345600 345600 345620 345620 5184000]
      | sbobj.Groups.Signals(3).YData = [0 0 10 10 0 0]
      | sbobj.Groups.TimeRange = [0 5184000]
  1 : Outport  Tag=STV Outport
  2 : Outport  Tag=STV Outport  Port=2
  3 : Outport  Tag=STV Outport  Port=3
  wires:
  Demux/1 -> 1/1
  Demux/2 -> 2/1
  Demux/3 -> 3/1
  FromWs/1 -> Demux/1

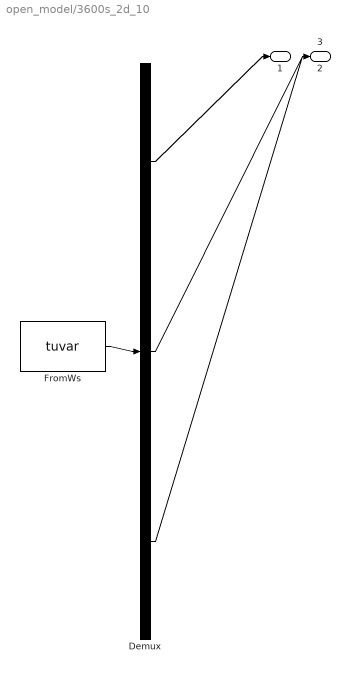
== system open_model/3600s_2d_10 ==
  Demux : Demux  Tag=STV Demux  Outputs=3
      settings: DisplayOption=none
  FromWs : FromWorkspace  Tag=STV FromWs  VariableName=tuvar
      SigBuilderData=|
      | common.afterFinalStr = 'Extrapolate'
      | common.sampleTime = 0
      | dataSet.timeRange = [0 864000]
      | dataSet.name = 'Group 1'
      | sbobj.Groups.Name = 'Group 1'
      | sbobj.Groups.Signals(1).Name = '1'
      | sbobj.Groups.Signals(1).XData = [0 3600 3600 864000]
      | sbobj.Groups.Signals(1).YData = [10 10 0 0]
      | sbobj.Groups.Signals(2).Name = '2'
      | sbobj.Groups.Signals(2).XData = [0 172800 172800 176400 176400 864000]
      | sbobj.Groups.Signals(2).YData = [0 0 10 10 0 0]
      | sbobj.Groups.Signals(3).Name = '3'
      | sbobj.Groups.Signals(3).XData = [0 345600 345600 349200 349200 864000]
      | sbobj.Groups.Signals(3).YData = [0 0 10 10 0 0]
      | sbobj.Groups.TimeRange = [0 864000]
  1 : Outport  Tag=STV Outport
  2 : Outport  Tag=STV Outport  Port=2
  3 : Outport  Tag=STV Outport  Port=3
  wires:
  Demux/1 -> 1/1
  Demux/2 -> 2/1
  Demux/3 -> 3/1
  FromWs/1 -> Demux/1

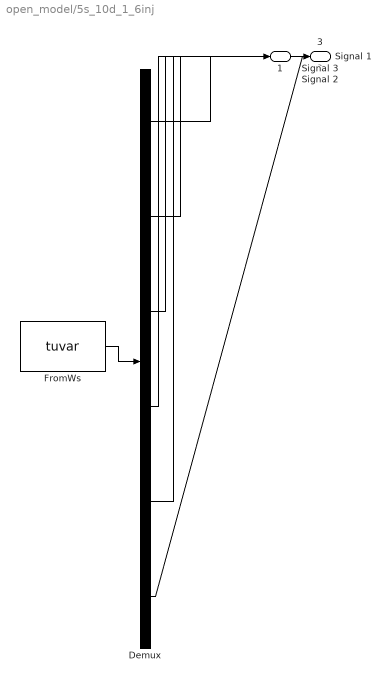
== system open_model/5s_10d_1_6inj ==
  Demux : Demux  Tag=STV Demux  Outputs=6
      settings: DisplayOption=none
  FromWs : FromWorkspace  Tag=STV FromWs  VariableName=tuvar
      SigBuilderData=|
      | common.afterFinalStr = 'Extrapolate'
      | common.sampleTime = 0
      | dataSet.timeRange = [0 5184000]
      | dataSet.name = 'Group 1'
      | sbobj.Groups.Name = 'Group 1'
      | sbobj.Groups.Signals(1).Name = '1'
      | sbobj.Groups.Signals(1).XData = [0 5 5 5184000]
      | sbobj.Groups.Signals(1).YData = [1 1 0 0]
      | sbobj.Groups.Signals(2).Name = '2'
      | sbobj.Groups.Signals(2).XData = [0 864000 864000 864005 864005 5184000]
      | sbobj.Groups.Signals(2).YData = [0 0 1 1 0 0]
      | sbobj.Groups.Signals(3).Name = '3'
      | sbobj.Groups.Signals(3).XData = [0 1728000 1728000 1728005 1728005 5184000]
      | sbobj.Groups.Signals(3).YData = [0 0 1 1 0 0]
      | sbobj.Groups.Signals(4).Name = 'Signal 1'
      | sbobj.Groups.Signals(4).XData = [0 2592000 2592000 2592005 2592005 5184000]
      | sbobj.Groups.Signals(4).YData = [0 0 1 1 0 0]
      | sbobj.Groups.Signals(5).Name = 'Signal 2'
      | sbobj.Groups.Signals(5).XData = [0 3456000 3456000 3456005 3456005 5184000]
      | sbobj.Groups.Signals(5).YData = [0 0 1 1 0 0]
      | sbobj.Groups.Signals(6).Name = 'Signal 3'
      | sbobj.Groups.Signals(6).XData = [0 4320000 4320000 4320005 4320005 5184000]
      | sbobj.Groups.Signals(6).YData = [0 0 1 1 0 0]
      | sbobj.Groups.TimeRange = [0 5184000]
  1 : Outport  Tag=STV Outport
  2 : Outport  Tag=STV Outport  Port=2
  3 : Outport  Tag=STV Outport  Port=3
  Signal 1 : Outport  Tag=STV Outport  Port=4
  Signal 2 : Outport  Tag=STV Outport  Port=5
  Signal 3 : Outport  Tag=STV Outport  Port=6
  wires:
  Demux/1 -> 1/1
  Demux/2 -> 2/1
  Demux/3 -> 3/1
  FromWs/1 -> Demux/1
  Demux/4 -> Signal 1/1
  Demux/5 -> Signal 2/1
  Demux/6 -> Signal 3/1

== system open_model/5s_10d_2_3inj ==
  Demux : Demux  Tag=STV Demux  Outputs=3
      settings: DisplayOption=none
  FromWs : FromWorkspace  Tag=STV FromWs  VariableName=tuvar
      SigBuilderData=|
      | common.afterFinalStr = 'Extrapolate'
      | common.sampleTime = 0
      | dataSet.timeRange = [0 2592000]
      | dataSet.name = 'Group 1'
      | sbobj.Groups.Name = 'Group 1'
      | sbobj.Groups.Signals(1).Name = '1'
      | sbobj.Groups.Signals(1).XData = [0 5 5 2592000]
      | sbobj.Groups.Signals(1).YData = [2 2 0 0]
      | sbobj.Groups.Signals(2).Name = '2'
      | sbobj.Groups.Signals(2).XData = [0 864000 864000 864005 864005 2592000]
      | sbobj.Groups.Signals(2).YData = [0 0 2 2 0 0]
      | sbobj.Groups.Signals(3).Name = 'Signal 1'
      | sbobj.Groups.Signals(3).XData = [0 1728000 1728000 1728005 1728005 2592000]
      | sbobj.Groups.Signals(3).YData = [0 0 2 2 0 0]
      | sbobj.Groups.TimeRange = [0 2592000]
  1 : Outport  Tag=STV Outport
  2 : Outport  Tag=STV Outport  Port=2
  Signal 1 : Outport  Tag=STV Outport  Port=3
  wires:
  FromWs/1 -> Demux/1
  Demux/2 -> 2/1
  Demux/1 -> 1/1
  Demux/3 -> Signal 1/1

== system open_model/5s_1d_2 ==
  Demux : Demux  Tag=STV Demux  Outputs=3
      settings: DisplayOption=none
  FromWs : FromWorkspace  Tag=STV FromWs  VariableName=tuvar
      SigBuilderData=|
      | common.afterFinalStr = 'Extrapolate'
      | common.sampleTime = 0
      | dataSet.timeRange = [0 864000]
      | dataSet.name = 'Group 1'
      | sbobj.Groups.Name = 'Group 1'
      | sbobj.Groups.Signals(1).Name = '1'
      | sbobj.Groups.Signals(1).XData = [0 5 5 864000]
      | sbobj.Groups.Signals(1).YData = [1 1 0 0]
      | sbobj.Groups.Signals(2).Name = '2'
      | sbobj.Groups.Signals(2).XData = [0 172800 172800 172805 172805 864000]
      | sbobj.Groups.Signals(2).YData = [0 0 2 2 0 0]
      | sbobj.Groups.Signals(3).Name = 'Signal 1'
      | sbobj.Groups.Signals(3).XData = [0 86400 86400 86405 86405 864000]
      | sbobj.Groups.Signals(3).YData = [0 0 2 2 0 0]
      | sbobj.Groups.TimeRange = [0 864000]
  1 : Outport  Tag=STV Outport
  2 : Outport  Tag=STV Outport  Port=2
  Signal 1 : Outport  Tag=STV Outport  Port=3
  wires:
  FromWs/1 -> Demux/1
  Demux/2 -> 2/1
  Demux/1 -> 1/1
  Demux/3 -> Signal 1/1

== system open_model/5s_2d_1 ==
  Demux : Demux  Tag=STV Demux  Outputs=1
      settings: DisplayOption=none
  FromWs : FromWorkspace  Tag=STV FromWs  VariableName=tuvar
      SigBuilderData=|
      | common.afterFinalStr = 'Extrapolate'
      | common.sampleTime = 0
      | dataSet.timeRange = [0 864000]
      | dataSet.name = 'Group 1'
      | sbobj.Groups.Name = 'Group 1'
      | sbobj.Groups.Signals.Name = '1'
      | sbobj.Groups.Signals.XData = [0 86400 86400 864000]
      | sbobj.Groups.Signals.YData = [0.0036 0.0036 0 0]
      | sbobj.Groups.TimeRange = [0 864000]
  1 : Outport  Tag=STV Outport
  wires:
  Demux/1 -> 1/1
  FromWs/1 -> Demux/1

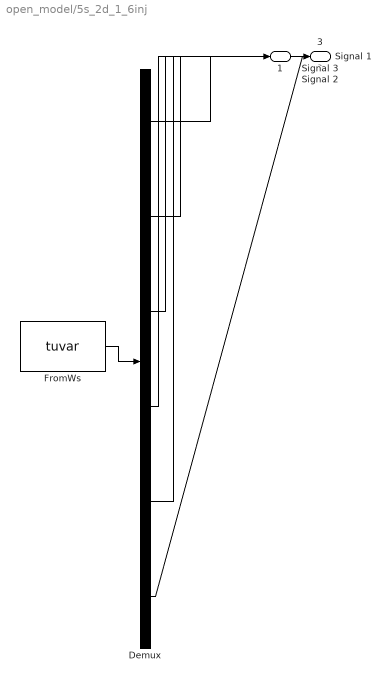
== system open_model/5s_2d_1_6inj ==
  Demux : Demux  Tag=STV Demux  Outputs=6
      settings: DisplayOption=none
  FromWs : FromWorkspace  Tag=STV FromWs  VariableName=tuvar
      SigBuilderData=|
      | common.afterFinalStr = 'Extrapolate'
      | common.sampleTime = 0
      | dataSet.timeRange = [0 1728000]
      | dataSet.name = 'Group 1'
      | sbobj.Groups.Name = 'Group 1'
      | sbobj.Groups.Signals(1).Name = '1'
      | sbobj.Groups.Signals(1).XData = [0 5 5 1728000]
      | sbobj.Groups.Signals(1).YData = [1 1 0 0]
      | sbobj.Groups.Signals(2).Name = '2'
      | sbobj.Groups.Signals(2).XData = [0 172800 172800 172805 172805 1728000]
      | sbobj.Groups.Signals(2).YData = [0 0 1 1 0 0]
      | sbobj.Groups.Signals(3).Name = '3'
      | sbobj.Groups.Signals(3).XData = [0 345600 345600 345605 345605 1728000]
      | sbobj.Groups.Signals(3).YData = [0 0 1 1 0 0]
      | sbobj.Groups.Signals(4).Name = 'Signal 1'
      | sbobj.Groups.Signals(4).XData = [0 518400 518400 518405 518405 1728000]
      | sbobj.Groups.Signals(4).YData = [0 0 1 1 0 0]
      | sbobj.Groups.Signals(5).Name = 'Signal 2'
      | sbobj.Groups.Signals(5).XData = [0 691200 691200 691205 691205 1728000]
      | sbobj.Groups.Signals(5).YData = [0 0 1 1 0 0]
      | sbobj.Groups.Signals(6).Name = 'Signal 3'
      | sbobj.Groups.Signals(6).XData = [0 864000 864000 864005 864005 1728000]
      | sbobj.Groups.Signals(6).YData = [0 0 1 1 0 0]
      | sbobj.Groups.TimeRange = [0 1728000]
  1 : Outport  Tag=STV Outport
  2 : Outport  Tag=STV Outport  Port=2
  3 : Outport  Tag=STV Outport  Port=3
  Signal 1 : Outport  Tag=STV Outport  Port=4
  Signal 2 : Outport  Tag=STV Outport  Port=5
  Signal 3 : Outport  Tag=STV Outport  Port=6
  wires:
  FromWs/1 -> Demux/1
  Demux/3 -> 3/1
  Demux/2 -> 2/1
  Demux/1 -> 1/1
  Demux/4 -> Signal 1/1
  Demux/5 -> Signal 2/1
  Demux/6 -> Signal 3/1

== system open_model/5s_2d_2_3inj ==
  Demux : Demux  Tag=STV Demux  Outputs=3
      settings: DisplayOption=none
  FromWs : FromWorkspace  Tag=STV FromWs  VariableName=tuvar
      SigBuilderData=|
      | common.afterFinalStr = 'Extrapolate'
      | common.sampleTime = 0
      | dataSet.timeRange = [0 864000]
      | dataSet.name = 'Group 1'
      | sbobj.Groups.Name = 'Group 1'
      | sbobj.Groups.Signals(1).Name = '1'
      | sbobj.Groups.Signals(1).XData = [0 5 5 864000]
      | sbobj.Groups.Signals(1).YData = [2 2 0 0]
      | sbobj.Groups.Signals(2).Name = '2'
      | sbobj.Groups.Signals(2).XData = [0 172800 172800 172805 172805 864000]
      | sbobj.Groups.Signals(2).YData = [0 0 2 2 0 0]
      | sbobj.Groups.Signals(3).Name = '3'
      | sbobj.Groups.Signals(3).XData = [0 345600 345600 345605 345605 864000]
      | sbobj.Groups.Signals(3).YData = [0 0 2 2 0 0]
      | sbobj.Groups.TimeRange = [0 864000]
  1 : Outport  Tag=STV Outport
  2 : Outport  Tag=STV Outport  Port=2
  3 : Outport  Tag=STV Outport  Port=3
  wires:
  FromWs/1 -> Demux/1
  Demux/3 -> 3/1
  Demux/2 -> 2/1
  Demux/1 -> 1/1

== system open_model/5s_2d_6 ==
  Demux : Demux  Tag=STV Demux  Outputs=1
      settings: DisplayOption=none
  FromWs : FromWorkspace  Tag=STV FromWs  VariableName=tuvar
      SigBuilderData=|
      | common.afterFinalStr = 'Extrapolate'
      | common.sampleTime = 0
      | dataSet.timeRange = [0 864000]
      | dataSet.name = 'Group 1'
      | sbobj.Groups.Name = 'Group 1'
      | sbobj.Groups.Signals.Name = '1'
      | sbobj.Groups.Signals.XData = [0 5 5 864000]
      | sbobj.Groups.Signals.YData = [6 6 0 0]
      | sbobj.Groups.TimeRange = [0 864000]
  1 : Outport  Tag=STV Outport
  wires:
  Demux/1 -> 1/1
  FromWs/1 -> Demux/1

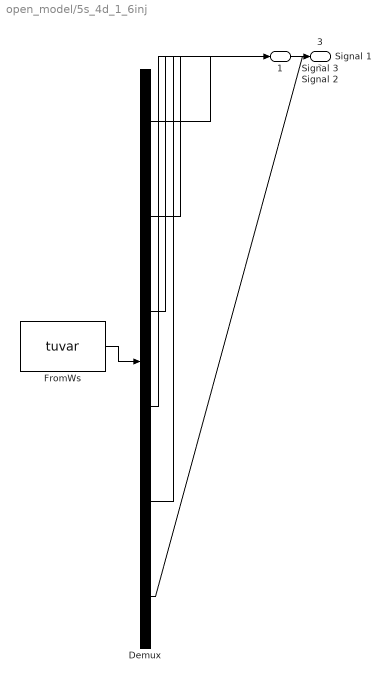
== system open_model/5s_4d_1_6inj ==
  Demux : Demux  Tag=STV Demux  Outputs=6
      settings: DisplayOption=none
  FromWs : FromWorkspace  Tag=STV FromWs  VariableName=tuvar
      SigBuilderData=|
      | common.afterFinalStr = 'Extrapolate'
      | common.sampleTime = 0
      | dataSet.timeRange = [0 5184000]
      | dataSet.name = 'Group 1'
      | sbobj.Groups.Name = 'Group 1'
      | sbobj.Groups.Signals(1).Name = '1'
      | sbobj.Groups.Signals(1).XData = [0 5 5 5184000]
      | sbobj.Groups.Signals(1).YData = [1 1 0 0]
      | sbobj.Groups.Signals(2).Name = '2'
      | sbobj.Groups.Signals(2).XData = [0 345600 345600 345605 345605 5184000]
      | sbobj.Groups.Signals(2).YData = [0 0 1 1 0 0]
      | sbobj.Groups.Signals(3).Name = '3'
      | sbobj.Groups.Signals(3).XData = [0 619200 619200 619205 619205 5184000]
      | sbobj.Groups.Signals(3).YData = [0 0 1 1 0 0]
      | sbobj.Groups.Signals(4).Name = 'Signal 1'
      | sbobj.Groups.Signals(4).XData = [0 1036800 1036800 1036805 1036805 5184000]
      | sbobj.Groups.Signals(4).YData = [0 0 1 1 0 0]
      | sbobj.Groups.Signals(5).Name = 'Signal 2'
      | sbobj.Groups.Signals(5).XData = [0 1382400 1382400 1382405 1382405 5184000]
      | sbobj.Groups.Signals(5).YData = [0 0 1 1 0 0]
      | sbobj.Groups.Signals(6).Name = 'Signal 3'
      | sbobj.Groups.Signals(6).XData = [0 1728000 1728000 1728005 1728005 5184000]
      | sbobj.Groups.Signals(6).YData = [0 0 1 1 0 0]
      | sbobj.Groups.TimeRange = [0 5184000]
  1 : Outport  Tag=STV Outport
  2 : Outport  Tag=STV Outport  Port=2
  3 : Outport  Tag=STV Outport  Port=3
  Signal 1 : Outport  Tag=STV Outport  Port=4
  Signal 2 : Outport  Tag=STV Outport  Port=5
  Signal 3 : Outport  Tag=STV Outport  Port=6
  wires:
  FromWs/1 -> Demux/1
  Demux/3 -> 3/1
  Demux/2 -> 2/1
  Demux/1 -> 1/1
  Demux/4 -> Signal 1/1
  Demux/5 -> Signal 2/1
  Demux/6 -> Signal 3/1

== system open_model/5s_4d_2_3inj ==
  Demux : Demux  Tag=STV Demux  Outputs=3
      settings: DisplayOption=none
  FromWs : FromWorkspace  Tag=STV FromWs  VariableName=tuvar
      SigBuilderData=|
      | common.afterFinalStr = 'Extrapolate'
      | common.sampleTime = 0
      | dataSet.timeRange = [0 2592000]
      | dataSet.name = 'Group 1'
      | sbobj.Groups.Name = 'Group 1'
      | sbobj.Groups.Signals(1).Name = '1'
      | sbobj.Groups.Signals(1).XData = [0 5 5 2592000]
      | sbobj.Groups.Signals(1).YData = [2 2 0 0]
      | sbobj.Groups.Signals(2).Name = '2'
      | sbobj.Groups.Signals(2).XData = [0 345600 345600 345605 345605 2592000]
      | sbobj.Groups.Signals(2).YData = [0 0 2 2 0 0]
      | sbobj.Groups.Signals(3).Name = '3'
      | sbobj.Groups.Signals(3).XData = [0 691200 691200 691205 691205 2592000]
      | sbobj.Groups.Signals(3).YData = [0 0 2 2 0 0]
      | sbobj.Groups.TimeRange = [0 2592000]
  1 : Outport  Tag=STV Outport
  2 : Outport  Tag=STV Outport  Port=2
  3 : Outport  Tag=STV Outport  Port=3
  wires:
  FromWs/1 -> Demux/1
  Demux/3 -> 3/1
  Demux/2 -> 2/1
  Demux/1 -> 1/1

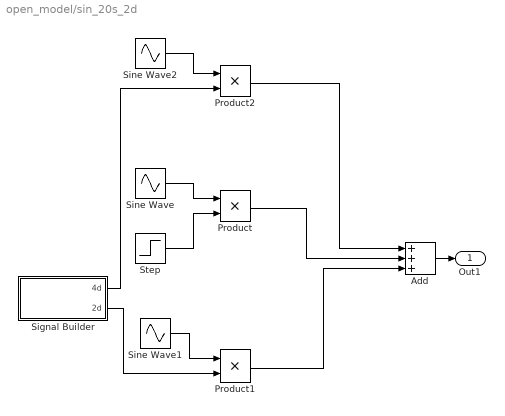
== system open_model/sin_20s_2d ==
  Add : Sum  Inputs=+++
  Product : Product
  Product1 : Product
  Product2 : Product
  Signal Builder : Subsystem  Tag=STV Subsys  LoadFcn=sigbuilder_block('load');  StartFcn=sigbuilder_block('start');  StopFcn=sigbuilder_block('stop');  ClipboardFcn=sigbuilder_block('clipboard');  mask(Sigbuilder block){tuvar=[0:10]}
      mask help: Simulink:masks:SigbuilderBlock_MD
      mask init:
      | if ~strcmp(get_param(bdroot(gcbh),'SimulationStatus'),'stopped') tuvar = sigbuilder_block('maskInit'); end
      settings: CopyFcn=sigbuilder_block('copy');  DeleteFcn=sigbuilder_block('delete');  ModelCloseFcn=sigbuilder_block('modelClose');  PreSaveFcn=sigbuilder_block('preSave');  PauseFcn=sigbuilder_block('pause');  ContinueFcn=sigbuilder_block('continue');  NameChangeFcn=sigbuilder_block('namechange');  OpenFcn=sigbuilder_block('open',[404 117.5 550.5 362.5 ]);  CloseFcn=sigbuilder_block('close');
      mask Display: plot(0, 0, 100, 100,[2, 2, 32, 32, 2], [68, 8, 8, 68, 68],[32, 2], [38, 38], [32, 19, 2],[53, 60, 44], [32, 17, 17, 2],[16, 16, 31, 31]);txt = getActiveGroup(gcbh);text(2, 100, txt,'verticalAlignment', 'top');
  Sine Wave : Sin  Amplitude=10  Frequency=pi/20  SampleTime=0
  Sine Wave1 : Sin  Amplitude=10  Frequency=pi/20  SampleTime=0
  Sine Wave2 : Sin  Amplitude=10  Frequency=pi/20  SampleTime=0
  Step : Step  Time=20  Before=1  After=0  SampleTime=0
  Out1 : Outport
  wires:
  Product1/1 -> Add/3
  Signal Builder/2(2d) -> Product1/2
  Signal Builder/1(4d) -> Product2/2
  Sine Wave2/1 -> Product2/1
  Product2/1 -> Add/1
  Sine Wave1/1 -> Product1/1
  Product/1 -> Add/2
  Step/1 -> Product/2
  Sine Wave/1 -> Product/1
  Add/1 -> Out1/1

== system open_model/sin_20s_2d/Signal Builder ==
  Demux : Demux  Tag=STV Demux  Outputs=2
      settings: DisplayOption=none
  FromWs : FromWorkspace  Tag=STV FromWs  VariableName=tuvar
      SigBuilderData=|
      | common.afterFinalStr = 'Extrapolate'
      | common.sampleTime = 0
      | dataSet.timeRange = [0 5184000]
      | dataSet.name = 'Group 1'
      | sbobj.Groups.Name = 'Group 1'
      | sbobj.Groups.Signals(1).Name = '4d'
      | sbobj.Groups.Signals(1).XData = [0 345600 345600 345620 345620 5184000]
      | sbobj.Groups.Signals(1).YData = [0 0 1 1 0 0]
      | sbobj.Groups.Signals(2).Name = '2d'
      | sbobj.Groups.Signals(2).XData = [0 172800 172800 172820 172820 5184000]
      | sbobj.Groups.Signals(2).YData = [0 0 1 1 0 0]
      | sbobj.Groups.TimeRange = [0 5184000]
  4d : Outport  Tag=STV Outport
  2d : Outport  Tag=STV Outport  Port=2
  wires:
  Demux/1 -> 4d/1
  FromWs/1 -> Demux/1
  Demux/2 -> 2d/1
